simulink model "untitled"  (R2024b)
settings: Solver=VariableStepAuto  StartTime=0.0  StopTime=10.0  RelTol=1e-3
undefined symbols (not defined in the file): Aero, Initial, Motor, Uav
settings Model: Creator=jski306  LastModifiedBy=jski306

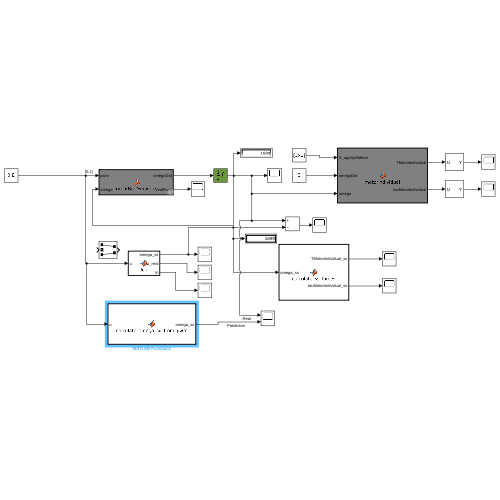
[thumbnail: Simulink's stored preview of the top-level diagram]
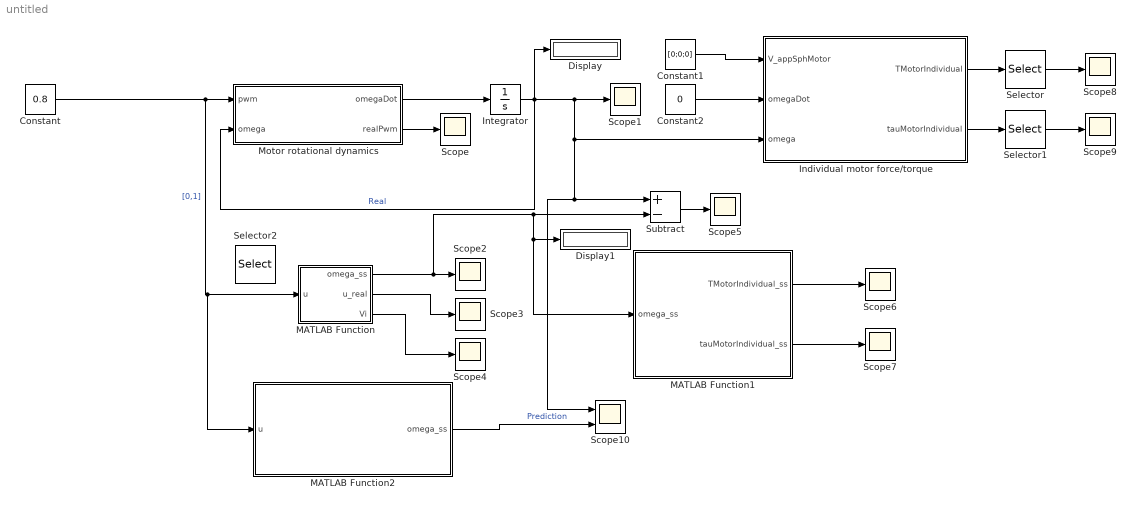
== system untitled ==
  Constant : Constant  Value=0.8
  Constant1 : Constant  Value=[0;0;0]
  Constant2 : Constant  Value=0
  Display : Display
  Display1 : Display
  Individual motor force/torque : MATLAB Function  TreatAsAtomicUnit=on
  Integrator : Integrator  InitialCondition=Initial.OMEGA  LimitOutput=on  LowerSaturationLimit=zeros(size(Initial.OMEGA))  ContinuousStateAttributes='omega'
  MATLAB Function : MATLAB Function  TreatAsAtomicUnit=on
  MATLAB Function1 : MATLAB Function  TreatAsAtomicUnit=on
  MATLAB Function2 : MATLAB Function  TreatAsAtomicUnit=on
  Motor rotational dynamics : MATLAB Function  TreatAsAtomicUnit=on
  Scope{,1..9} (10 alike) : Scope
  Scope10 : Scope  NumInputPorts=2
  Selector : Selector  NumberOfDimensions=2  InputPortWidth=3  IndexOptions=Index vector (dialog),Index vector (dialog)  Indices=[1 3],1  OutputSizes=1,1
  Selector1 : Selector  NumberOfDimensions=2  InputPortWidth=3  IndexOptions=Index vector (dialog),Index vector (dialog)  Indices=[1 3],1  OutputSizes=1,1
  Selector2 : Selector  InputPortWidth=3  IndexOptions=Index vector (dialog)  Indices=[1 3]  OutputSizes=1
  Subtract : Sum  Inputs=+-
  wires:
  Integrator/1 -> Display/1, Individual motor force/torque/3(omega), Scope10/1, Subtract/1, Scope1/1, Motor rotational dynamics/2(omega)  "Real"
  Motor rotational dynamics/1(omegaDot) -> Integrator/1
  Motor rotational dynamics/2(realPwm) -> Scope/1
  Constant/1 -> MATLAB Function2/1(u), MATLAB Function/1(u), Motor rotational dynamics/1(pwm)  "[0,1]"
  MATLAB Function/1(omega_ss) -> Display1/1, MATLAB Function1/1(omega_ss), Subtract/2, Scope2/1
  MATLAB Function/2(u_real) -> Scope3/1
  MATLAB Function/3(Vi) -> Scope4/1
  Subtract/1 -> Scope5/1
  MATLAB Function1/1(TMotorIndividual_ss) -> Scope6/1
  MATLAB Function1/2(tauMotorIndividual_ss) -> Scope7/1
  Constant1/1 -> Individual motor force/torque/1(V_appSphMotor)
  Constant2/1 -> Individual motor force/torque/2(omegaDot)
  Individual motor force/torque/1(TMotorIndividual) -> Selector/1
  Individual motor force/torque/2(tauMotorIndividual) -> Selector1/1
  Selector/1 -> Scope8/1
  Selector1/1 -> Scope9/1
  MATLAB Function2/1(omega_ss) -> Scope10/2  "Prediction"

== matlab function untitled/MATLAB Function ==
  data: u input; omega_ss output; u_real output; Motor parameter; Vi output
function [omega_ss,u_real,Vi] = fcn(u, Motor)
%CALCOMEGASS_U Calculate steady-state motor speed from normalised command U
%   U      - Normalised PWM command in [0, 1]
%   Motor  - Struct containing motor parameters (same fields as in motorRotDynamics)
%
% Output:
%   omega_ss - Steady-state rotor speed (rad/s)

% Extract first element of each motor parameter array
Kt   = Motor.K_T(1);
Ke   = Motor.K_E(1);
R    = Motor.R(1);
Ctau = Motor.C_TAU(1);
mv   = Motor.volt_slope(1);
Voff = Motor.Volt_offset(1);
I0   = Motor.I_0(1);
u_max  = Motor.pwm_max(1);
u_min  = Motor.pwm_min(1);

u_real = u * (u_max - u_min) + u_min;
% Input voltage
% Coefficients of the quadratic equation: A*omega^2 + B*omega + C = 0
A = Ctau;
B = (Kt * Ke ) / R;

% The constant term 'C' is a function of the input PWM
Vi = mv * u + Voff;
C = - (Kt / R) * (Vi - I0  * R);

% Calculate the discriminant of the quadratic formula
discriminant = B^2 - 4*A*C;

% The steady-state speed is 0 if the discriminant is negative, meaning
% the input voltage is not enough to overcome the no-load current draw.
if discriminant < 0
    omega_ss = 0;
else
    % Solve using the quadratic formula, taking the positive root for
    % the physically meaningful solution (forward rotation).
    omega_ss = (-B + sqrt(discriminant)) / (2*A);
end

== matlab function untitled/Motor rotational dynamics ==
  data: pwm input; omegaDot output; omega input; realPwm output; Motor parameter
function [omegaDot, realPwm]  = motorRotDynamics( pwm, omega, Motor )
%#codegen
%MOTORROTDYNAMICS Implement brushless DC motor model.
%   Based on permanent magnet DC motor model.
%   Written: J.X.J. Bannwarth

    % Normalised PWM (in [0, 1] range) to voltage conversion
    Vi = Motor.volt_slope.*pwm + Motor.Volt_offset;

    % Motor dynamics
    omegaDot = (1./Motor.I_R_ZZ') .* ( ...
        (Motor.K_T./Motor.R) .* ( Vi - Motor.I_0.*Motor.R - omega.*Motor.K_E ) - ...
        Motor.C_TAU.*omega.^2 );

    % Compute real PWM (in us) from normalised PWM
    realPwm = pwm.*(Motor.pwm_max-Motor.pwm_min) + Motor.pwm_min;
end

== matlab function untitled/MATLAB Function1 ==
  data: omega_ss input; TMotorIndividual_ss output; tauMotorIndividual_ss output; Motor parameter; Uav parameter; Aero parameter
function [TMotorIndividual_ss, tauMotorIndividual_ss] = calculate_ss_forces( ...
    omega_ss, Motor, Uav, Aero )
%#codegen
% CALCULATE_SS_FORCES Computes the steady-state thrust and torque vectors
% for a single motor under hover conditions (U=0, alpha=0, beta=0).
%
% This function implements the simplified analytical expressions derived from
% the 'motorIndividual' dynamics. It is intended to be used for validation
% by comparing its output to the full dynamic model at steady state.

%% Extract Parameters for the First Motor
% This function is designed to calculate for a single motor. We will use
% the parameters corresponding to the first motor (index 1).

rho_air         = Uav.RHO_AIR;
prop_diameter   = Uav.D_PROP(1);
prop_area       = Uav.A_PROP(1);
rotor_direction = Uav.ROTOR_DIRECTION(1);

% Aerodynamic coefficients
p_z3 = Aero.Cz3P.coefs(1);

% Motor-specific coefficients
C_tau = Motor.C_TAU(1);

%% Calculate Steady-State Thrust (TMotorIndividual_ss)

% Under hover conditions, side forces (Txy) are zero.
% The thrust (Tz) is calculated from the simplified expression.
Tz_ss = -0.5 * rho_air * p_z3 * (prop_diameter^2) * prop_area * (omega_ss^2);

% Assemble the 3x1 thrust vector
TMotorIndividual_ss = [0; 0; Tz_ss];

%% Calculate Steady-State Torque (tauMotorIndividual_ss)

% Under hover conditions, aerodynamic moments (Mxy) are zero.
% The torque (tau_z) is the reaction torque from aerodynamic drag.
tau_z_ss = -rotor_direction * C_tau * (omega_ss^2);

% Assemble the 3x1 torque vector
tauMotorIndividual_ss = [0; 0; tau_z_ss];

end

== matlab function untitled/Individual motor force//torque ==
  data: V_appSphMotor input; omegaDot input; omega input; TMotorIndividual output; Motor parameter; Uav parameter; tauMotorIndividual output; Aero parameter
function [TMotorIndividual, tauMotorIndividual] = motorIndividual( ...
    V_appSphMotor, omegaDot, omega, Motor, Uav, Aero )
%#codegen
    alpha = V_appSphMotor(2,:);
    beta  = V_appSphMotor(1,:);
    U     = V_appSphMotor(3,:);
    
    % Make assertions to avoid code generation errors
    %assert(Uav.N_ROTORS < 16);

    %% Thrusts
    % Concatenated motor force/torque vectors in respective motor frame
    % eg. TMotor = [TMotor1, TMotor2, ..., TMotorN]
    % where: - N is the number of rotors
    %        - TMotorx (x ∈ [1,2,...,N]) is the thrust generated by motor x in
    %          its own frame of reference
    % For basic thrust model:
    % TMotorIndividual = [ zeros(2, Uav.N_ROTORS);
    %                      K * (omega'.^2) ];

% %Cx1 for rotor
% p = Aero.Cx1P.coefs;
% Cx1 = p(:,1)' .* cos(alpha) + p(:,2)' .* cos(3*alpha) + p(:,3)' .* cos(7*alpha);
% 
% %Cz1 for rotor
% p = Aero.Cz1P.coefs;
% Cz1 = p(:,1)' .* sin(alpha) + p(:,2)';

%Cx2 for rotor
p = Aero.Cx2P.coefs;
lambda = omega' .* Uav.D_PROP' ./ ( 2 * U );
Cx2 = p(:,1)' .* ( 1 - exp(-p(:,2)'.*lambda) ) .* cos(alpha) + ...
    p(:,3)' .* ( 1 - exp(-p(:,4)'.*lambda) ) .* cos(3*alpha);

%Cz2 for rotor
p = Aero.Cz2P.coefs;
Cz2 = p(:,1)' .* sin(alpha) + p(:,2)' .* ( 1 - exp(-p(:,3)'.*lambda) ) .* sin(3*alpha) + ...
    p(:,4)';

%Cz3 for rotor
Cz3 = Aero.Cz3P.coefs';

%Rotor Thrust
% Tz = 0.5 .* Uav.RHO_AIR .* (Cz1) .* U .* U .* Uav.A_PROP' + ...
%     0.5 .* Uav.RHO_AIR .* omega'.^2 .* (Cz3) .* Uav.D_PROP'.^2 .* Uav.A_PROP' + ...
%     0.5 .* Uav.RHO_AIR .* (Cz2) .* U .*  omega' .* Uav.D_PROP' .* Uav.A_PROP';
Tz = -0.5 .* Uav.RHO_AIR .* omega'.^2 .* (Cz3) .* Uav.D_PROP'.^2 .* Uav.A_PROP' + ...
    -0.5 .* Uav.RHO_AIR .* (Cz2) .* U .*  omega' .* Uav.D_PROP' .* Uav.A_PROP';

%Rotor side loads
% Txy = 0.5 .* Uav.RHO_AIR .* (Cx1) .* U .* U .* Uav.A_PROP' + ...
%     0.5 .* Uav.RHO_AIR .* (Cx2) .* U .* omega' .* Uav.D_PROP' .* Uav.D_PROP';
Txy = -0.5 .* Uav.RHO_AIR .* (Cx2) .* U .* omega' .* Uav.D_PROP' .* Uav.A_PROP';
TMotorIndividual = [ Txy.*cos(beta); Txy.*sin(beta); Tz ];

%% Moments
% %CM1 for rotor
% p = Aero.CM1P.coefs;
% CM1 = p(:,1)' .* cos(alpha) + p(:,2)' .* cos(3*alpha) + p(:,3)' .* sin(2*alpha);

%CM2 for rotor
p = Aero.CM2P.coefs;
CM2 = p(:,1)' .* ( 1 - exp(-p(:,2)'.*lambda) ) .* cos(alpha) + ...
    p(:,3)' .* ( 1 - exp(-p(:,4)'.*lambda) ) .* sin(2*alpha);

%Moments
% Mxy = 0.5 .* Uav.RHO_AIR .* (CM1) .* U .* U .* Uav.A_PROP' .* Uav.D_PROP' ...
%     + 0.5 .* Uav.RHO_AIR .* U .* omega' .* CM2 .* Uav.A_PROP' .* Uav.D_PROP'.^2;
Mxy = 0.5 .* Uav.RHO_AIR .* U .* omega' .* CM2 .* Uav.A_PROP' .* Uav.D_PROP'.^2;
tauMotorIndividual = [ Mxy.*sin(beta); Mxy.*cos(beta);
    -Uav.ROTOR_DIRECTION .* ( Motor.C_TAU' .* omega'.^2 + Motor.I_R_ZZ .* omegaDot' ) ];
end

== matlab function untitled/MATLAB Function2 ==
  data: u input; omega_ss output; Motor parameter
function omega_ss = calculate_omega_sq_from_pwm(u, Motor)
%calculate_omega_sq_from_pwm Solves for omega^2 for all motors using a for loop.
%   This version iterates through each motor, applying the exact scalar
%   logic that has been verified to work correctly.

    % Determine the number of motors from the input PWM vector
    N_motors = numel(u);
    
    % Pre-allocate the output vector for speed
    omega_ss = zeros(N_motors, 1);

    % Loop through each motor
    for i = 1:N_motors
        % --- 1. Extract scalar parameters for the current motor ---
        Kt   = Motor.K_T(i);
        Ke   = Motor.K_E(i);
        R    = Motor.R(i);
        Ctau = Motor.C_TAU(i);
        mv   = Motor.volt_slope(i);
        Voff = Motor.Volt_offset(i);
        I0   = Motor.I_0(i);
        u_max  = Motor.pwm_max(i);
        u_min  = Motor.pwm_min(i);

        u_real = u * (u_max - u_min) + u_min;
        
        % Input voltage
        % Coefficients of the quadratic equation: A*omega^2 + B*omega + C = 0
        A = Ctau;
        B = (Kt * Ke ) / R;


        % The constant term 'C' is a function of the input PWM
        Vi = mv * u(i) + Voff;
        C = - (Kt / R) * (Vi - I0  * R);
        
        % Calculate the discriminant of the quadratic formula
        discriminant = B^2 - 4*A*C;
        
        % The steady-state speed is 0 if the discriminant is negative, meaning
        % the input voltage is not enough to overcome the no-load current draw.
        if discriminant < 0
            omega_ss(i) = 0;
        else
            % Solve using the quadratic formula, taking the positive root for
            % the physically meaningful solution (forward rotation).
            omega_ss(i) = (-B + sqrt(discriminant)) / (2*A);
        end

    end

end
